simulink model "vlokvo_m"  (Simulink 7.9)
settings: Solver=ode45  SolverMode=SingleTasking  StartTime=0.0  StopTime=999999  MaxStep=10  RelTol=1e-3  AbsTol=1e-3
values from neighbouring files (symbols this model uses):
  U = st_Varia('LongNames')    [vlokvo_i.m]
  x0 = zeros(P.NumCel,1)    [vlokvo_i.m]    (also in vlokvo_s.m = x0)
undefined symbols (not defined in the file or in its folder): B
settings Model: Creator=M.Sparnaaij  LastModifiedBy=M.Sparnaaij
settings DataIOCC: LimitDataPoints=off  SaveOutput=off  SaveTime=off  SignalLoggingName=sigsOut
settings OptimizationCC: BooleanDataType=off
settings DebuggingCC: SaveWithParameterizedLinksMsg=none  SignalResolutionControl=TryResolveAllWithWarning  SolverPrmCheckMsg=none  MultiTaskDSMMsg=warning  MultiTaskCondExecSysMsg=none  StrictBusMsg=None
settings HardwareCC: TargetUnknown=on
settings RTWCC: IncludeERTFirstTime=on
settings GRTTargetCC: CombineOutputUpdateFcns=off  GRTInterface=on

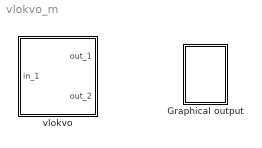
== system vlokvo_m ==
  Graphical output : Subsystem
      settings: OpenFcn=vlokvo_g
      mask Display:
      | plot(0,0,100,100,[80,20,20],[20,20,80],[80,69,60,52,45,39,33,28,24,20],[65,65,64,61,57,52,45,37,30,20])
      | disp('');
      | text(100,100,'vlokvo', 'horizontalAlignment', 'right', 'verticalAlignment', 'top');
  vlokvo : Subsystem  Description=This model calculates the removal of suspended solids with a flocculation reactor.
      mask init:
      | filenaam='.\StimelaData\Flocculation.mat';
      | 
      | [Pn,Fn,Fext]=Fileprop(filenaam);
      | 
      | errstr = st_UniqName(filenaam,'filenaam=''','SubSystem','OpenFcn');
      | if errstr, error([errstr 'The filename "' filenaam '" is already in use. Choose a different filename.']), end
      | 
      | P = vlokvo_p(filenaam);
      | [B,x0,U]=vlokvo_i(filenaam);
      settings: OpenFcn=|
      | filenaam='.\StimelaData\Flocculation.mat';
      | st_ParameterInput('init',gcb,filenaam,'vlokvo');
      mask Display:
      | plot(0,0,100,100,[80,80,20,20],[80,20,20,80],[80,20],[70,70],[50,50],[90,40],[50,61,65,67,69,70,70,69,67,65,61,50],[40,46,47,47,45,42,38,35,33,33,34,40],[50,39,35,33,31,30,30,31,33,35,39,50],[40,46,47,47,45,42,38,35,33,33,34,40])
      | disp('')
      | text(50,50,'vlokvo', 'horizontalAlignment', 'center', 'verticalAlignment', 'middle');
      | text(50,0,Fn, 'horizontalAlignment', 'center', 'verticalAlignment', 'base');

== system vlokvo_m/Graphical output ==
  note: plotten

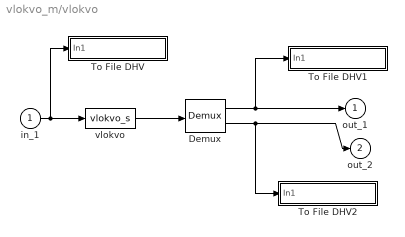
== system vlokvo_m/vlokvo ==
  in_1 : Inport
  Demux : Demux  Outputs=[U.Number B.Measurements]
  To File DHV : Subsystem  mask(To File DHV){naam=[filenaam(1:length(filenaam)-4) '_in.sti']}
      mask prompts: naam "Naam van bestand"
      mask init:
      | set_param([gcb '/To File'],'Filename',naam);
      mask Display: disp(naam)
  To File DHV1 : Subsystem  mask(To File DHV){naam=[filenaam(1:length(filenaam)-4) '_out.sti']}
      mask prompts: naam "Naam van bestand"
      mask init:
      | set_param([gcb '/To File'],'Filename',naam);
      mask Display: disp(naam)
  To File DHV2 : Subsystem  mask(To File DHV){naam=[filenaam(1:length(filenaam)-4) '_EM.sti']}
      mask prompts: naam "Naam van bestand"
      mask init:
      | set_param([gcb '/To File'],'Filename',naam);
      mask Display: disp(naam)
  vlokvo : S-Function  FunctionName=vlokvo_s  Parameters=B,x0,U,P  EnableBusSupport=off
  out_1 : Outport  InitialOutput=0
  out_2 : Outport  Port=2  InitialOutput=0
  wires:
  in_1/1 -> To File DHV/1(In1), vlokvo/1
  Demux/2 -> To File DHV2/1(In1), out_2/1
  Demux/1 -> To File DHV1/1(In1), out_1/1
  vlokvo/1 -> Demux/1

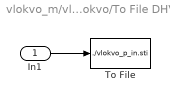
== system vlokvo_m/vlokvo/To File DHV ==
  In1 : Inport
  To File : ToFile  Filename=./vlokvo_p_in.sti  MatrixName=vlokvoin
  wires:
  In1/1 -> To File/1

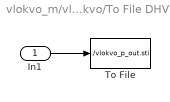
== system vlokvo_m/vlokvo/To File DHV1 ==
  In1 : Inport
  To File : ToFile  Filename=./vlokvo_p_out.sti  MatrixName=vlokvoout
  wires:
  In1/1 -> To File/1

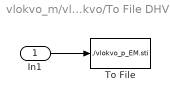
== system vlokvo_m/vlokvo/To File DHV2 ==
  In1 : Inport
  To File : ToFile  Filename=./vlokvo_p_EM.sti  MatrixName=vlokvoEM
  wires:
  In1/1 -> To File/1
